simulink model "HotAirBalloon_NonlinearModel_R2015a_step"  (R2017b)
settings: Solver=ode4  StartTime=0.0  StopTime=SIM_TIME  FixedStep=STEP_SIZE  RelTol=1e-3
undefined symbols (not defined in the file or in its folder): b, c, f, g, M, Ta0, tau1, V, x0
settings Model: Creator=eh  LastModifiedBy=lasse
settings DataIOCC: LimitDataPoints=on  SaveFormat=Array  SignalLoggingSaveFormat=ModelDataLogs
settings OptimizationCC: ExpressionDepthLimit=2147483647  InitFltsAndDblsToZero=on  LifeSpan=inf
settings DebuggingCC: SaveWithParameterizedLinksMsg=none  UnderspecifiedInitializationDetection=Classic  MergeDetectMultiDrivingBlocksExec=none  SignalResolutionControl=TryResolveAllWithWarning  SolverPrmCheckMsg=warning  MultiTaskDSMMsg=warning  MultiTaskCondExecSysMsg=none  FcnCallInpInsideContextMsg=warning  StateNameClashWarn=warning  SFUnexpectedBacktrackingDiag=warning  SFNoUnconditionalDefaultTransitionDiag=warning  SFExecutionAtInitializationDiag=none
settings HardwareCC: ProdBitPerPointer=32  ProdBitPerSizeT=32  ProdBitPerPtrDiffT=32  ProdLargestAtomicFloat=None  ProdIntDivRoundTo=Undefined  ProdEndianess=Unspecified  ProdWordSize=32  ProdHWDeviceType=32-bit Generic
settings ModelReferenceCC: PropagateSignalLabelsOutOfModel=off
settings CodeAppCC: StateflowObjectComments=on
settings GRTTargetCC: TargetFcnLib=ansi_tfl_tmw.mat  TargetLangStandard=C89/C90 (ANSI)  CombineOutputUpdateFcns=off  GRTInterface=on
settings ConfigComp: CovMetricSettings=dw  CovHtmlReporting=on  CovSaveCumulativeToWorkspaceVar=on  CovSaveSingleToWorkspaceVar=on  CovExternalEMLEnable=off

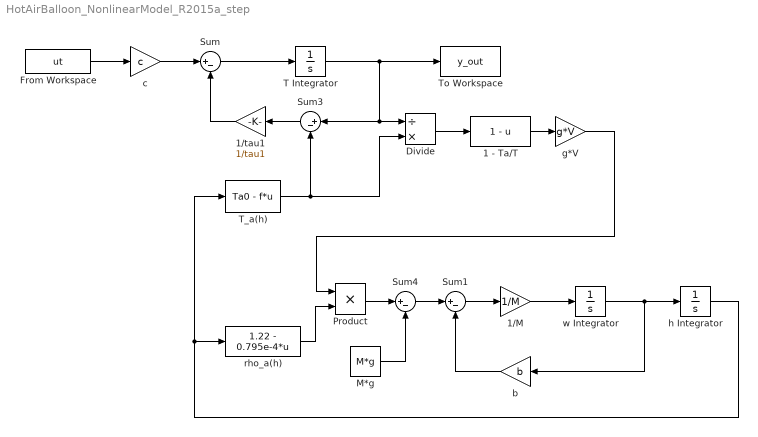
== system HotAirBalloon_NonlinearModel_R2015a_step ==
  1 - Ta/T : Fcn  Expr=1 - u
  1/M : Gain  Gain=1/M
  1/tau1 : Gain  Gain=1/tau1
  Divide : Product  Inputs=/*
  From Workspace : FromWorkspace  VariableName=ut  SampleTime=0
  M*g : Constant  Value=M*g
  Product : Product  RndMeth=Zero
  Sum{,1,3..4} (4 alike) : Sum  Inputs=|+-
  T Integrator : Integrator  Priority=1  InitialCondition=x0(1)
  T_a(h) : Fcn  Expr=Ta0 - f*u
  To Workspace : ToWorkspace  VariableName=y_out  SaveFormat=Timeseries  SampleTime=-1
  b : Gain  Gain=b
  c : Gain  Gain=c
  g*V : Gain  Gain=g*V
  h Integrator : Integrator  Priority=3  InitialCondition=x0(3)
  rho_a(h) : Fcn  Expr=1.22 - 0.795e-4*u
  w Integrator : Integrator  Priority=2  InitialCondition=x0(2)
  wires:
  c/1 -> Sum/1
  T Integrator/1 -> To Workspace/1, Divide/1, Sum3/1
  w Integrator/1 -> h Integrator/1, b/1
  Sum/1 -> T Integrator/1
  Sum3/1 -> 1/tau1/1
  1/tau1/1 -> Sum/2
  T_a(h)/1 -> Sum3/2, Divide/2
  Sum1/1 -> 1/M/1
  b/1 -> Sum1/2
  Product/1 -> Sum4/1
  Sum4/1 -> Sum1/1
  M*g/1 -> Sum4/2
  Divide/1 -> 1 - Ta/T/1
  1 - Ta/T/1 -> g*V/1
  rho_a(h)/1 -> Product/2
  From Workspace/1 -> c/1
  g*V/1 -> Product/1
  h Integrator/1 -> rho_a(h)/1, T_a(h)/1
  1/M/1 -> w Integrator/1
